simulink model "HMI_2L_StMdXX_Rsp"  (R2018b)
settings: Solver=FixedStepDiscrete  StartTime=0.0  StopTime=10.0  FixedStep=0.01  RelTol=1e-3
undefined symbols (not defined in the file or in its folder): KeSMSuRspStatHldTm_Val, SrcReqTp1
libraries: RspLib x20
(part 1 of 2)
settings Model: Creator=sn2xws  LastModifiedBy=sn2xws
settings DataIOCC: SaveFormat=StructureWithTime
settings OptimizationCC: DefaultParameterBehavior=Inlined  EnhancedBackFolding=on  PassReuseOutputArgsAs=Individual arguments  ZeroExternalMemoryAtStartup=off  ZeroInternalMemoryAtStartup=off  OptimizeBlockOrder=speed  DifferentSizesBufferReuse=on  OptimizationCustomize=off
settings DebuggingCC: ParameterTunabilityLossMsg=error
settings ModelReferenceCC: ModelReferenceNumInstancesAllowed=Single
settings SFSimCC: MATLABDynamicMemAlloc=off
settings RTWCC: SystemTargetFile=autosar.tlc  GenCodeOnly=on  TemplateMakefile=ert_default_tmf  Description=AUTOSAR  GenerateReport=on  IncludeHyperlinkInReport=on  LaunchReport=on  GenerateTraceInfo=on  GenerateTraceReport=on  GenerateTraceReportSl=on  GenerateTraceReportSf=on  GenerateTraceReportEml=on
settings CodeAppCC: ForceParamTrailComments=on  IgnoreCustomStorageClasses=off  OperatorAnnotations=on  SimulinkDataObjDesc=on  SFDataObjDesc=on  InsertBlockDesc=on
settings STFCustomTargetCC: TargetLangStandard=C99 (ISO)  MultiwordLength=256  ParMdlRefBuildCompliant=on  CompOptLevelCompliant=on  IncludeMdlTerminateFcn=off  CombineOutputUpdateFcns=on  SuppressErrorStatus=on  ERTCustomFileBanners=on  SupportNonFinite=off  SupportComplex=off  SupportContinuousTime=off  SupportNonInlinedSFcns=off  RemoveResetFunc=on  MATLABClassNameForMDSCustomization=Simulink.SoftwareTarget.ERTCustomization  AutosarCompliant=on  UseToolchainInfoCompliant=on  LookupTableObjectStructAxisOrder=2,1,3,4,...  LUTObjectStructOrderEvenSpacing=Size,Table,Breakpoints  SystemTargetFile=autosar.tlc
settings ERTTargetCC: TargetLangStandard=C99 (ISO)  ConcurrentExecutionCompliant=off  IncludeMdlTerminateFcn=off  SuppressErrorStatus=on  SupportNonFinite=off  SupportComplex=off  ModelStepFunctionPrototypeControlCompliant=off  CPPClassGenCompliant=off  AutosarCompliant=on  LookupTableObjectStructAxisOrder=2,1,3,4,...  LUTObjectStructOrderEvenSpacing=Size,Table,Breakpoints  InlinedParameterPlacement=NonHierarchical  ERTCustomFileTemplate=example_file_process.tlc

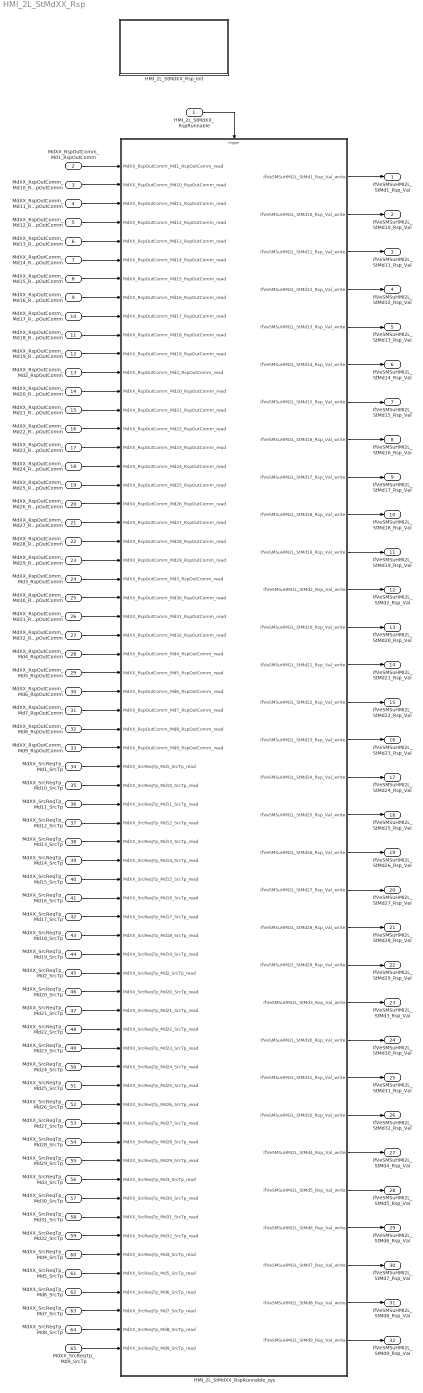
== system HMI_2L_StMdXX_Rsp ==
  HMI_2L_StMdXX_RspRunnable : Inport  SampleTime=0.01  OutputFunctionCall=on
  MdXX_RspOutComm_Md1_RspOutComm : Inport  Port=2  OutDataTypeStr=uint8  PortDimensions=1
  MdXX_RspOutComm_Md10_RspOutComm : Inport  Port=3  OutDataTypeStr=uint8  PortDimensions=1
  MdXX_RspOutComm_Md11_RspOutComm : Inport  Port=4  OutDataTypeStr=uint8  PortDimensions=1
  MdXX_RspOutComm_Md12_RspOutComm : Inport  Port=5  OutDataTypeStr=uint8  PortDimensions=1
  MdXX_RspOutComm_Md13_RspOutComm : Inport  Port=6  OutDataTypeStr=uint8  PortDimensions=1
  MdXX_RspOutComm_Md14_RspOutComm : Inport  Port=7  OutDataTypeStr=uint8  PortDimensions=1
  MdXX_RspOutComm_Md15_RspOutComm : Inport  Port=8  OutDataTypeStr=uint8  PortDimensions=1
  MdXX_RspOutComm_Md16_RspOutComm : Inport  Port=9  OutDataTypeStr=uint8  PortDimensions=1
  MdXX_RspOutComm_Md17_RspOutComm : Inport  Port=10  OutDataTypeStr=uint8  PortDimensions=1
  MdXX_RspOutComm_Md18_RspOutComm : Inport  Port=11  OutDataTypeStr=uint8  PortDimensions=1
  MdXX_RspOutComm_Md19_RspOutComm : Inport  Port=12  OutDataTypeStr=uint8  PortDimensions=1
  MdXX_RspOutComm_Md2_RspOutComm : Inport  Port=13  OutDataTypeStr=uint8  PortDimensions=1
  MdXX_RspOutComm_Md20_RspOutComm : Inport  Port=14  OutDataTypeStr=uint8  PortDimensions=1
  MdXX_RspOutComm_Md21_RspOutComm : Inport  Port=15  OutDataTypeStr=uint8  PortDimensions=1
  MdXX_RspOutComm_Md22_RspOutComm : Inport  Port=16  OutDataTypeStr=uint8  PortDimensions=1
  MdXX_RspOutComm_Md23_RspOutComm : Inport  Port=17  OutDataTypeStr=uint8  PortDimensions=1
  MdXX_RspOutComm_Md24_RspOutComm : Inport  Port=18  OutDataTypeStr=uint8  PortDimensions=1
  MdXX_RspOutComm_Md25_RspOutComm : Inport  Port=19  OutDataTypeStr=uint8  PortDimensions=1
  MdXX_RspOutComm_Md26_RspOutComm : Inport  Port=20  OutDataTypeStr=uint8  PortDimensions=1
  MdXX_RspOutComm_Md27_RspOutComm : Inport  Port=21  OutDataTypeStr=uint8  PortDimensions=1
  MdXX_RspOutComm_Md28_RspOutComm : Inport  Port=22  OutDataTypeStr=uint8  PortDimensions=1
  MdXX_RspOutComm_Md29_RspOutComm : Inport  Port=23  OutDataTypeStr=uint8  PortDimensions=1
  MdXX_RspOutComm_Md3_RspOutComm : Inport  Port=24  OutDataTypeStr=uint8  PortDimensions=1
  MdXX_RspOutComm_Md30_RspOutComm : Inport  Port=25  OutDataTypeStr=uint8  PortDimensions=1
  MdXX_RspOutComm_Md31_RspOutComm : Inport  Port=26  OutDataTypeStr=uint8  PortDimensions=1
  MdXX_RspOutComm_Md32_RspOutComm : Inport  Port=27  OutDataTypeStr=uint8  PortDimensions=1
  MdXX_RspOutComm_Md4_RspOutComm : Inport  Port=28  OutDataTypeStr=uint8  PortDimensions=1
  MdXX_RspOutComm_Md5_RspOutComm : Inport  Port=29  OutDataTypeStr=uint8  PortDimensions=1
  MdXX_RspOutComm_Md6_RspOutComm : Inport  Port=30  OutDataTypeStr=uint8  PortDimensions=1
  MdXX_RspOutComm_Md7_RspOutComm : Inport  Port=31  OutDataTypeStr=uint8  PortDimensions=1
  MdXX_RspOutComm_Md8_RspOutComm : Inport  Port=32  OutDataTypeStr=uint8  PortDimensions=1
  MdXX_RspOutComm_Md9_RspOutComm : Inport  Port=33  OutDataTypeStr=uint8  PortDimensions=1
  MdXX_SrcReqTp_Md1_SrcTp : Inport  Port=34  OutDataTypeStr=Enum: SrcReqTp1  PortDimensions=1
  MdXX_SrcReqTp_Md10_SrcTp : Inport  Port=35  OutDataTypeStr=Enum: SrcReqTp1  PortDimensions=1
  MdXX_SrcReqTp_Md11_SrcTp : Inport  Port=36  OutDataTypeStr=Enum: SrcReqTp1  PortDimensions=1
  MdXX_SrcReqTp_Md12_SrcTp : Inport  Port=37  OutDataTypeStr=Enum: SrcReqTp1  PortDimensions=1
  MdXX_SrcReqTp_Md13_SrcTp : Inport  Port=38  OutDataTypeStr=Enum: SrcReqTp1  PortDimensions=1
  MdXX_SrcReqTp_Md14_SrcTp : Inport  Port=39  OutDataTypeStr=Enum: SrcReqTp1  PortDimensions=1
  MdXX_SrcReqTp_Md15_SrcTp : Inport  Port=40  OutDataTypeStr=Enum: SrcReqTp1  PortDimensions=1
  MdXX_SrcReqTp_Md16_SrcTp : Inport  Port=41  OutDataTypeStr=Enum: SrcReqTp1  PortDimensions=1
  MdXX_SrcReqTp_Md17_SrcTp : Inport  Port=42  OutDataTypeStr=Enum: SrcReqTp1  PortDimensions=1
  MdXX_SrcReqTp_Md18_SrcTp : Inport  Port=43  OutDataTypeStr=Enum: SrcReqTp1  PortDimensions=1
  MdXX_SrcReqTp_Md19_SrcTp : Inport  Port=44  OutDataTypeStr=Enum: SrcReqTp1  PortDimensions=1
  MdXX_SrcReqTp_Md2_SrcTp : Inport  Port=45  OutDataTypeStr=Enum: SrcReqTp1  PortDimensions=1
  MdXX_SrcReqTp_Md20_SrcTp : Inport  Port=46  OutDataTypeStr=Enum: SrcReqTp1  PortDimensions=1
  MdXX_SrcReqTp_Md21_SrcTp : Inport  Port=47  OutDataTypeStr=Enum: SrcReqTp1  PortDimensions=1
  MdXX_SrcReqTp_Md22_SrcTp : Inport  Port=48  OutDataTypeStr=Enum: SrcReqTp1  PortDimensions=1
  MdXX_SrcReqTp_Md23_SrcTp : Inport  Port=49  OutDataTypeStr=Enum: SrcReqTp1  PortDimensions=1
  MdXX_SrcReqTp_Md24_SrcTp : Inport  Port=50  OutDataTypeStr=Enum: SrcReqTp1  PortDimensions=1
  MdXX_SrcReqTp_Md25_SrcTp : Inport  Port=51  OutDataTypeStr=Enum: SrcReqTp1  PortDimensions=1
  MdXX_SrcReqTp_Md26_SrcTp : Inport  Port=52  OutDataTypeStr=Enum: SrcReqTp1  PortDimensions=1
  MdXX_SrcReqTp_Md27_SrcTp : Inport  Port=53  OutDataTypeStr=Enum: SrcReqTp1  PortDimensions=1
  MdXX_SrcReqTp_Md28_SrcTp : Inport  Port=54  OutDataTypeStr=Enum: SrcReqTp1  PortDimensions=1
  MdXX_SrcReqTp_Md29_SrcTp : Inport  Port=55  OutDataTypeStr=Enum: SrcReqTp1  PortDimensions=1
  MdXX_SrcReqTp_Md3_SrcTp : Inport  Port=56  OutDataTypeStr=Enum: SrcReqTp1  PortDimensions=1
  MdXX_SrcReqTp_Md30_SrcTp : Inport  Port=57  OutDataTypeStr=Enum: SrcReqTp1  PortDimensions=1
  MdXX_SrcReqTp_Md31_SrcTp : Inport  Port=58  OutDataTypeStr=Enum: SrcReqTp1  PortDimensions=1
  MdXX_SrcReqTp_Md32_SrcTp : Inport  Port=59  OutDataTypeStr=Enum: SrcReqTp1  PortDimensions=1
  MdXX_SrcReqTp_Md4_SrcTp : Inport  Port=60  OutDataTypeStr=Enum: SrcReqTp1  PortDimensions=1
  MdXX_SrcReqTp_Md5_SrcTp : Inport  Port=61  OutDataTypeStr=Enum: SrcReqTp1  PortDimensions=1
  MdXX_SrcReqTp_Md6_SrcTp : Inport  Port=62  OutDataTypeStr=Enum: SrcReqTp1  PortDimensions=1
  MdXX_SrcReqTp_Md7_SrcTp : Inport  Port=63  OutDataTypeStr=Enum: SrcReqTp1  PortDimensions=1
  MdXX_SrcReqTp_Md8_SrcTp : Inport  Port=64  OutDataTypeStr=Enum: SrcReqTp1  PortDimensions=1
  MdXX_SrcReqTp_Md9_SrcTp : Inport  Port=65  OutDataTypeStr=Enum: SrcReqTp1  PortDimensions=1
  HMI_2L_StMdXX_RspRunnable_sys : Subsystem
  HMI_2L_StMdXX_Rsp_Init : Subsystem
  IfVeSMSuHMI2L_StMd1_Rsp_Val : Outport  OutDataTypeStr=uint8  PortDimensions=1
  IfVeSMSuHMI2L_StMd10_Rsp_Val : Outport  Port=2  OutDataTypeStr=uint8  PortDimensions=1
  IfVeSMSuHMI2L_StMd11_Rsp_Val : Outport  Port=3  OutDataTypeStr=uint8  PortDimensions=1
  IfVeSMSuHMI2L_StMd12_Rsp_Val : Outport  Port=4  OutDataTypeStr=uint8  PortDimensions=1
  IfVeSMSuHMI2L_StMd13_Rsp_Val : Outport  Port=5  OutDataTypeStr=uint8  PortDimensions=1
  IfVeSMSuHMI2L_StMd14_Rsp_Val : Outport  Port=6  OutDataTypeStr=uint8  PortDimensions=1
  IfVeSMSuHMI2L_StMd15_Rsp_Val : Outport  Port=7  OutDataTypeStr=uint8  PortDimensions=1
  IfVeSMSuHMI2L_StMd16_Rsp_Val : Outport  Port=8  OutDataTypeStr=uint8  PortDimensions=1
  IfVeSMSuHMI2L_StMd17_Rsp_Val : Outport  Port=9  OutDataTypeStr=uint8  PortDimensions=1
  IfVeSMSuHMI2L_StMd18_Rsp_Val : Outport  Port=10  OutDataTypeStr=uint8  PortDimensions=1
  IfVeSMSuHMI2L_StMd19_Rsp_Val : Outport  Port=11  OutDataTypeStr=uint8  PortDimensions=1
  IfVeSMSuHMI2L_StMd2_Rsp_Val : Outport  Port=12  OutDataTypeStr=uint8  PortDimensions=1
  IfVeSMSuHMI2L_StMd20_Rsp_Val : Outport  Port=13  OutDataTypeStr=uint8  PortDimensions=1
  IfVeSMSuHMI2L_StMd21_Rsp_Val : Outport  Port=14  OutDataTypeStr=uint8  PortDimensions=1
  IfVeSMSuHMI2L_StMd22_Rsp_Val : Outport  Port=15  OutDataTypeStr=uint8  PortDimensions=1
  IfVeSMSuHMI2L_StMd23_Rsp_Val : Outport  Port=16  OutDataTypeStr=uint8  PortDimensions=1
  IfVeSMSuHMI2L_StMd24_Rsp_Val : Outport  Port=17  OutDataTypeStr=uint8  PortDimensions=1
  IfVeSMSuHMI2L_StMd25_Rsp_Val : Outport  Port=18  OutDataTypeStr=uint8  PortDimensions=1
  IfVeSMSuHMI2L_StMd26_Rsp_Val : Outport  Port=19  OutDataTypeStr=uint8  PortDimensions=1
  IfVeSMSuHMI2L_StMd27_Rsp_Val : Outport  Port=20  OutDataTypeStr=uint8  PortDimensions=1
  IfVeSMSuHMI2L_StMd28_Rsp_Val : Outport  Port=21  OutDataTypeStr=uint8  PortDimensions=1
  IfVeSMSuHMI2L_StMd29_Rsp_Val : Outport  Port=22  OutDataTypeStr=uint8  PortDimensions=1
  IfVeSMSuHMI2L_StMd3_Rsp_Val : Outport  Port=23  OutDataTypeStr=uint8  PortDimensions=1
  IfVeSMSuHMI2L_StMd30_Rsp_Val : Outport  Port=24  OutDataTypeStr=uint8  PortDimensions=1
  IfVeSMSuHMI2L_StMd31_Rsp_Val : Outport  Port=25  OutDataTypeStr=uint8  PortDimensions=1
  IfVeSMSuHMI2L_StMd32_Rsp_Val : Outport  Port=26  OutDataTypeStr=uint8  PortDimensions=1
  IfVeSMSuHMI2L_StMd4_Rsp_Val : Outport  Port=27  OutDataTypeStr=uint8  PortDimensions=1
  IfVeSMSuHMI2L_StMd5_Rsp_Val : Outport  Port=28  OutDataTypeStr=uint8  PortDimensions=1
  IfVeSMSuHMI2L_StMd6_Rsp_Val : Outport  Port=29  OutDataTypeStr=uint8  PortDimensions=1
  IfVeSMSuHMI2L_StMd7_Rsp_Val : Outport  Port=30  OutDataTypeStr=uint8  PortDimensions=1
  IfVeSMSuHMI2L_StMd8_Rsp_Val : Outport  Port=31  OutDataTypeStr=uint8  PortDimensions=1
  IfVeSMSuHMI2L_StMd9_Rsp_Val : Outport  Port=32  OutDataTypeStr=uint8  PortDimensions=1
  wires:
  MdXX_RspOutComm_Md1_RspOutComm/1 -> HMI_2L_StMdXX_RspRunnable_sys/1(MdXX_RspOutComm_Md1_RspOutComm_read)
  MdXX_RspOutComm_Md10_RspOutComm/1 -> HMI_2L_StMdXX_RspRunnable_sys/2(MdXX_RspOutComm_Md10_RspOutComm_read)
  MdXX_RspOutComm_Md11_RspOutComm/1 -> HMI_2L_StMdXX_RspRunnable_sys/3(MdXX_RspOutComm_Md11_RspOutComm_read)
  MdXX_RspOutComm_Md12_RspOutComm/1 -> HMI_2L_StMdXX_RspRunnable_sys/4(MdXX_RspOutComm_Md12_RspOutComm_read)
  MdXX_RspOutComm_Md13_RspOutComm/1 -> HMI_2L_StMdXX_RspRunnable_sys/5(MdXX_RspOutComm_Md13_RspOutComm_read)
  MdXX_RspOutComm_Md14_RspOutComm/1 -> HMI_2L_StMdXX_RspRunnable_sys/6(MdXX_RspOutComm_Md14_RspOutComm_read)
  MdXX_RspOutComm_Md15_RspOutComm/1 -> HMI_2L_StMdXX_RspRunnable_sys/7(MdXX_RspOutComm_Md15_RspOutComm_read)
  MdXX_RspOutComm_Md16_RspOutComm/1 -> HMI_2L_StMdXX_RspRunnable_sys/8(MdXX_RspOutComm_Md16_RspOutComm_read)
  MdXX_RspOutComm_Md17_RspOutComm/1 -> HMI_2L_StMdXX_RspRunnable_sys/9(MdXX_RspOutComm_Md17_RspOutComm_read)
  MdXX_RspOutComm_Md18_RspOutComm/1 -> HMI_2L_StMdXX_RspRunnable_sys/10(MdXX_RspOutComm_Md18_RspOutComm_read)
  MdXX_RspOutComm_Md19_RspOutComm/1 -> HMI_2L_StMdXX_RspRunnable_sys/11(MdXX_RspOutComm_Md19_RspOutComm_read)
  MdXX_RspOutComm_Md2_RspOutComm/1 -> HMI_2L_StMdXX_RspRunnable_sys/12(MdXX_RspOutComm_Md2_RspOutComm_read)
  MdXX_RspOutComm_Md20_RspOutComm/1 -> HMI_2L_StMdXX_RspRunnable_sys/13(MdXX_RspOutComm_Md20_RspOutComm_read)
  MdXX_RspOutComm_Md21_RspOutComm/1 -> HMI_2L_StMdXX_RspRunnable_sys/14(MdXX_RspOutComm_Md21_RspOutComm_read)
  MdXX_RspOutComm_Md22_RspOutComm/1 -> HMI_2L_StMdXX_RspRunnable_sys/15(MdXX_RspOutComm_Md22_RspOutComm_read)
  MdXX_RspOutComm_Md23_RspOutComm/1 -> HMI_2L_StMdXX_RspRunnable_sys/16(MdXX_RspOutComm_Md23_RspOutComm_read)
  MdXX_RspOutComm_Md24_RspOutComm/1 -> HMI_2L_StMdXX_RspRunnable_sys/17(MdXX_RspOutComm_Md24_RspOutComm_read)
  MdXX_RspOutComm_Md25_RspOutComm/1 -> HMI_2L_StMdXX_RspRunnable_sys/18(MdXX_RspOutComm_Md25_RspOutComm_read)
  MdXX_RspOutComm_Md26_RspOutComm/1 -> HMI_2L_StMdXX_RspRunnable_sys/19(MdXX_RspOutComm_Md26_RspOutComm_read)
  MdXX_RspOutComm_Md27_RspOutComm/1 -> HMI_2L_StMdXX_RspRunnable_sys/20(MdXX_RspOutComm_Md27_RspOutComm_read)
  MdXX_RspOutComm_Md28_RspOutComm/1 -> HMI_2L_StMdXX_RspRunnable_sys/21(MdXX_RspOutComm_Md28_RspOutComm_read)
  MdXX_RspOutComm_Md29_RspOutComm/1 -> HMI_2L_StMdXX_RspRunnable_sys/22(MdXX_RspOutComm_Md29_RspOutComm_read)
  MdXX_RspOutComm_Md3_RspOutComm/1 -> HMI_2L_StMdXX_RspRunnable_sys/23(MdXX_RspOutComm_Md3_RspOutComm_read)
  MdXX_RspOutComm_Md30_RspOutComm/1 -> HMI_2L_StMdXX_RspRunnable_sys/24(MdXX_RspOutComm_Md30_RspOutComm_read)
  MdXX_RspOutComm_Md31_RspOutComm/1 -> HMI_2L_StMdXX_RspRunnable_sys/25(MdXX_RspOutComm_Md31_RspOutComm_read)
  MdXX_RspOutComm_Md32_RspOutComm/1 -> HMI_2L_StMdXX_RspRunnable_sys/26(MdXX_RspOutComm_Md32_RspOutComm_read)
  MdXX_RspOutComm_Md4_RspOutComm/1 -> HMI_2L_StMdXX_RspRunnable_sys/27(MdXX_RspOutComm_Md4_RspOutComm_read)
  MdXX_RspOutComm_Md5_RspOutComm/1 -> HMI_2L_StMdXX_RspRunnable_sys/28(MdXX_RspOutComm_Md5_RspOutComm_read)
  MdXX_RspOutComm_Md6_RspOutComm/1 -> HMI_2L_StMdXX_RspRunnable_sys/29(MdXX_RspOutComm_Md6_RspOutComm_read)
  MdXX_RspOutComm_Md7_RspOutComm/1 -> HMI_2L_StMdXX_RspRunnable_sys/30(MdXX_RspOutComm_Md7_RspOutComm_read)
  MdXX_RspOutComm_Md8_RspOutComm/1 -> HMI_2L_StMdXX_RspRunnable_sys/31(MdXX_RspOutComm_Md8_RspOutComm_read)
  MdXX_RspOutComm_Md9_RspOutComm/1 -> HMI_2L_StMdXX_RspRunnable_sys/32(MdXX_RspOutComm_Md9_RspOutComm_read)
  MdXX_SrcReqTp_Md1_SrcTp/1 -> HMI_2L_StMdXX_RspRunnable_sys/33(MdXX_SrcReqTp_Md1_SrcTp_read)
  MdXX_SrcReqTp_Md10_SrcTp/1 -> HMI_2L_StMdXX_RspRunnable_sys/34(MdXX_SrcReqTp_Md10_SrcTp_read)
  MdXX_SrcReqTp_Md11_SrcTp/1 -> HMI_2L_StMdXX_RspRunnable_sys/35(MdXX_SrcReqTp_Md11_SrcTp_read)
  MdXX_SrcReqTp_Md12_SrcTp/1 -> HMI_2L_StMdXX_RspRunnable_sys/36(MdXX_SrcReqTp_Md12_SrcTp_read)
  MdXX_SrcReqTp_Md13_SrcTp/1 -> HMI_2L_StMdXX_RspRunnable_sys/37(MdXX_SrcReqTp_Md13_SrcTp_read)
  MdXX_SrcReqTp_Md14_SrcTp/1 -> HMI_2L_StMdXX_RspRunnable_sys/38(MdXX_SrcReqTp_Md14_SrcTp_read)
  MdXX_SrcReqTp_Md15_SrcTp/1 -> HMI_2L_StMdXX_RspRunnable_sys/39(MdXX_SrcReqTp_Md15_SrcTp_read)
  MdXX_SrcReqTp_Md16_SrcTp/1 -> HMI_2L_StMdXX_RspRunnable_sys/40(MdXX_SrcReqTp_Md16_SrcTp_read)
  MdXX_SrcReqTp_Md17_SrcTp/1 -> HMI_2L_StMdXX_RspRunnable_sys/41(MdXX_SrcReqTp_Md17_SrcTp_read)
  MdXX_SrcReqTp_Md18_SrcTp/1 -> HMI_2L_StMdXX_RspRunnable_sys/42(MdXX_SrcReqTp_Md18_SrcTp_read)
  MdXX_SrcReqTp_Md19_SrcTp/1 -> HMI_2L_StMdXX_RspRunnable_sys/43(MdXX_SrcReqTp_Md19_SrcTp_read)
  MdXX_SrcReqTp_Md2_SrcTp/1 -> HMI_2L_StMdXX_RspRunnable_sys/44(MdXX_SrcReqTp_Md2_SrcTp_read)
  MdXX_SrcReqTp_Md20_SrcTp/1 -> HMI_2L_StMdXX_RspRunnable_sys/45(MdXX_SrcReqTp_Md20_SrcTp_read)
  MdXX_SrcReqTp_Md21_SrcTp/1 -> HMI_2L_StMdXX_RspRunnable_sys/46(MdXX_SrcReqTp_Md21_SrcTp_read)
  MdXX_SrcReqTp_Md22_SrcTp/1 -> HMI_2L_StMdXX_RspRunnable_sys/47(MdXX_SrcReqTp_Md22_SrcTp_read)
  MdXX_SrcReqTp_Md23_SrcTp/1 -> HMI_2L_StMdXX_RspRunnable_sys/48(MdXX_SrcReqTp_Md23_SrcTp_read)
  MdXX_SrcReqTp_Md24_SrcTp/1 -> HMI_2L_StMdXX_RspRunnable_sys/49(MdXX_SrcReqTp_Md24_SrcTp_read)
  MdXX_SrcReqTp_Md25_SrcTp/1 -> HMI_2L_StMdXX_RspRunnable_sys/50(MdXX_SrcReqTp_Md25_SrcTp_read)
  MdXX_SrcReqTp_Md26_SrcTp/1 -> HMI_2L_StMdXX_RspRunnable_sys/51(MdXX_SrcReqTp_Md26_SrcTp_read)
  MdXX_SrcReqTp_Md27_SrcTp/1 -> HMI_2L_StMdXX_RspRunnable_sys/52(MdXX_SrcReqTp_Md27_SrcTp_read)
  MdXX_SrcReqTp_Md28_SrcTp/1 -> HMI_2L_StMdXX_RspRunnable_sys/53(MdXX_SrcReqTp_Md28_SrcTp_read)
  MdXX_SrcReqTp_Md29_SrcTp/1 -> HMI_2L_StMdXX_RspRunnable_sys/54(MdXX_SrcReqTp_Md29_SrcTp_read)
  MdXX_SrcReqTp_Md3_SrcTp/1 -> HMI_2L_StMdXX_RspRunnable_sys/55(MdXX_SrcReqTp_Md3_SrcTp_read)
  MdXX_SrcReqTp_Md30_SrcTp/1 -> HMI_2L_StMdXX_RspRunnable_sys/56(MdXX_SrcReqTp_Md30_SrcTp_read)
  MdXX_SrcReqTp_Md31_SrcTp/1 -> HMI_2L_StMdXX_RspRunnable_sys/57(MdXX_SrcReqTp_Md31_SrcTp_read)
  MdXX_SrcReqTp_Md32_SrcTp/1 -> HMI_2L_StMdXX_RspRunnable_sys/58(MdXX_SrcReqTp_Md32_SrcTp_read)
  MdXX_SrcReqTp_Md4_SrcTp/1 -> HMI_2L_StMdXX_RspRunnable_sys/59(MdXX_SrcReqTp_Md4_SrcTp_read)
  MdXX_SrcReqTp_Md5_SrcTp/1 -> HMI_2L_StMdXX_RspRunnable_sys/60(MdXX_SrcReqTp_Md5_SrcTp_read)
  MdXX_SrcReqTp_Md6_SrcTp/1 -> HMI_2L_StMdXX_RspRunnable_sys/61(MdXX_SrcReqTp_Md6_SrcTp_read)
  MdXX_SrcReqTp_Md7_SrcTp/1 -> HMI_2L_StMdXX_RspRunnable_sys/62(MdXX_SrcReqTp_Md7_SrcTp_read)
  MdXX_SrcReqTp_Md8_SrcTp/1 -> HMI_2L_StMdXX_RspRunnable_sys/63(MdXX_SrcReqTp_Md8_SrcTp_read)
  MdXX_SrcReqTp_Md9_SrcTp/1 -> HMI_2L_StMdXX_RspRunnable_sys/64(MdXX_SrcReqTp_Md9_SrcTp_read)
  HMI_2L_StMdXX_RspRunnable_sys/1(IfVeSMSuHMI2L_StMd1_Rsp_Val_write) -> IfVeSMSuHMI2L_StMd1_Rsp_Val/1
  HMI_2L_StMdXX_RspRunnable_sys/2(IfVeSMSuHMI2L_StMd10_Rsp_Val_write) -> IfVeSMSuHMI2L_StMd10_Rsp_Val/1
  HMI_2L_StMdXX_RspRunnable_sys/3(IfVeSMSuHMI2L_StMd11_Rsp_Val_write) -> IfVeSMSuHMI2L_StMd11_Rsp_Val/1
  HMI_2L_StMdXX_RspRunnable_sys/4(IfVeSMSuHMI2L_StMd12_Rsp_Val_write) -> IfVeSMSuHMI2L_StMd12_Rsp_Val/1
  HMI_2L_StMdXX_RspRunnable_sys/5(IfVeSMSuHMI2L_StMd13_Rsp_Val_write) -> IfVeSMSuHMI2L_StMd13_Rsp_Val/1
  HMI_2L_StMdXX_RspRunnable_sys/6(IfVeSMSuHMI2L_StMd14_Rsp_Val_write) -> IfVeSMSuHMI2L_StMd14_Rsp_Val/1
  HMI_2L_StMdXX_RspRunnable_sys/7(IfVeSMSuHMI2L_StMd15_Rsp_Val_write) -> IfVeSMSuHMI2L_StMd15_Rsp_Val/1
  HMI_2L_StMdXX_RspRunnable_sys/8(IfVeSMSuHMI2L_StMd16_Rsp_Val_write) -> IfVeSMSuHMI2L_StMd16_Rsp_Val/1
  HMI_2L_StMdXX_RspRunnable_sys/9(IfVeSMSuHMI2L_StMd17_Rsp_Val_write) -> IfVeSMSuHMI2L_StMd17_Rsp_Val/1
  HMI_2L_StMdXX_RspRunnable_sys/10(IfVeSMSuHMI2L_StMd18_Rsp_Val_write) -> IfVeSMSuHMI2L_StMd18_Rsp_Val/1
  HMI_2L_StMdXX_RspRunnable_sys/11(IfVeSMSuHMI2L_StMd19_Rsp_Val_write) -> IfVeSMSuHMI2L_StMd19_Rsp_Val/1
  HMI_2L_StMdXX_RspRunnable_sys/12(IfVeSMSuHMI2L_StMd2_Rsp_Val_write) -> IfVeSMSuHMI2L_StMd2_Rsp_Val/1
  HMI_2L_StMdXX_RspRunnable_sys/13(IfVeSMSuHMI2L_StMd20_Rsp_Val_write) -> IfVeSMSuHMI2L_StMd20_Rsp_Val/1
  HMI_2L_StMdXX_RspRunnable_sys/14(IfVeSMSuHMI2L_StMd21_Rsp_Val_write) -> IfVeSMSuHMI2L_StMd21_Rsp_Val/1
  HMI_2L_StMdXX_RspRunnable_sys/15(IfVeSMSuHMI2L_StMd22_Rsp_Val_write) -> IfVeSMSuHMI2L_StMd22_Rsp_Val/1
  HMI_2L_StMdXX_RspRunnable_sys/16(IfVeSMSuHMI2L_StMd23_Rsp_Val_write) -> IfVeSMSuHMI2L_StMd23_Rsp_Val/1
  HMI_2L_StMdXX_RspRunnable_sys/17(IfVeSMSuHMI2L_StMd24_Rsp_Val_write) -> IfVeSMSuHMI2L_StMd24_Rsp_Val/1
  HMI_2L_StMdXX_RspRunnable_sys/18(IfVeSMSuHMI2L_StMd25_Rsp_Val_write) -> IfVeSMSuHMI2L_StMd25_Rsp_Val/1
  HMI_2L_StMdXX_RspRunnable_sys/19(IfVeSMSuHMI2L_StMd26_Rsp_Val_write) -> IfVeSMSuHMI2L_StMd26_Rsp_Val/1
  HMI_2L_StMdXX_RspRunnable_sys/20(IfVeSMSuHMI2L_StMd27_Rsp_Val_write) -> IfVeSMSuHMI2L_StMd27_Rsp_Val/1
  HMI_2L_StMdXX_RspRunnable_sys/21(IfVeSMSuHMI2L_StMd28_Rsp_Val_write) -> IfVeSMSuHMI2L_StMd28_Rsp_Val/1
  HMI_2L_StMdXX_RspRunnable_sys/22(IfVeSMSuHMI2L_StMd29_Rsp_Val_write) -> IfVeSMSuHMI2L_StMd29_Rsp_Val/1
  HMI_2L_StMdXX_RspRunnable_sys/23(IfVeSMSuHMI2L_StMd3_Rsp_Val_write) -> IfVeSMSuHMI2L_StMd3_Rsp_Val/1
  HMI_2L_StMdXX_RspRunnable_sys/24(IfVeSMSuHMI2L_StMd30_Rsp_Val_write) -> IfVeSMSuHMI2L_StMd30_Rsp_Val/1
  HMI_2L_StMdXX_RspRunnable_sys/25(IfVeSMSuHMI2L_StMd31_Rsp_Val_write) -> IfVeSMSuHMI2L_StMd31_Rsp_Val/1
  HMI_2L_StMdXX_RspRunnable_sys/26(IfVeSMSuHMI2L_StMd32_Rsp_Val_write) -> IfVeSMSuHMI2L_StMd32_Rsp_Val/1
  HMI_2L_StMdXX_RspRunnable_sys/27(IfVeSMSuHMI2L_StMd4_Rsp_Val_write) -> IfVeSMSuHMI2L_StMd4_Rsp_Val/1
  HMI_2L_StMdXX_RspRunnable_sys/28(IfVeSMSuHMI2L_StMd5_Rsp_Val_write) -> IfVeSMSuHMI2L_StMd5_Rsp_Val/1
  HMI_2L_StMdXX_RspRunnable_sys/29(IfVeSMSuHMI2L_StMd6_Rsp_Val_write) -> IfVeSMSuHMI2L_StMd6_Rsp_Val/1
  HMI_2L_StMdXX_RspRunnable_sys/30(IfVeSMSuHMI2L_StMd7_Rsp_Val_write) -> IfVeSMSuHMI2L_StMd7_Rsp_Val/1
  HMI_2L_StMdXX_RspRunnable_sys/31(IfVeSMSuHMI2L_StMd8_Rsp_Val_write) -> IfVeSMSuHMI2L_StMd8_Rsp_Val/1
  HMI_2L_StMdXX_RspRunnable_sys/32(IfVeSMSuHMI2L_StMd9_Rsp_Val_write) -> IfVeSMSuHMI2L_StMd9_Rsp_Val/1
  HMI_2L_StMdXX_RspRunnable/1 -> HMI_2L_StMdXX_RspRunnable_sys/Trigger

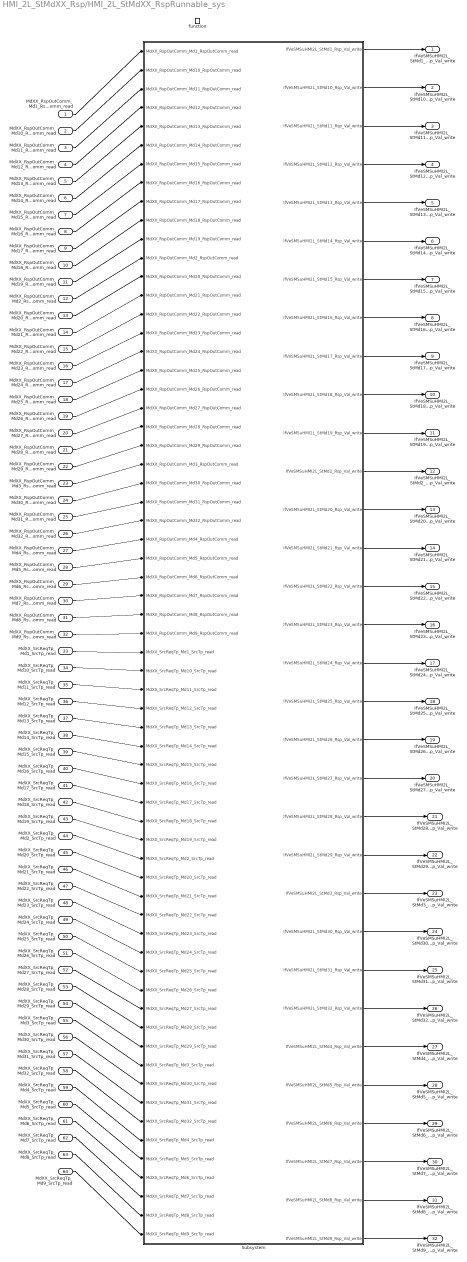
== system HMI_2L_StMdXX_Rsp/HMI_2L_StMdXX_RspRunnable_sys ==
  MdXX_RspOutComm_Md1_RspOutComm_read : Inport
  MdXX_RspOutComm_Md10_RspOutComm_read : Inport  Port=2
  MdXX_RspOutComm_Md11_RspOutComm_read : Inport  Port=3
  MdXX_RspOutComm_Md12_RspOutComm_read : Inport  Port=4
  MdXX_RspOutComm_Md13_RspOutComm_read : Inport  Port=5
  MdXX_RspOutComm_Md14_RspOutComm_read : Inport  Port=6
  MdXX_RspOutComm_Md15_RspOutComm_read : Inport  Port=7
  MdXX_RspOutComm_Md16_RspOutComm_read : Inport  Port=8
  MdXX_RspOutComm_Md17_RspOutComm_read : Inport  Port=9
  MdXX_RspOutComm_Md18_RspOutComm_read : Inport  Port=10
  MdXX_RspOutComm_Md19_RspOutComm_read : Inport  Port=11
  MdXX_RspOutComm_Md2_RspOutComm_read : Inport  Port=12
  MdXX_RspOutComm_Md20_RspOutComm_read : Inport  Port=13
  MdXX_RspOutComm_Md21_RspOutComm_read : Inport  Port=14
  MdXX_RspOutComm_Md22_RspOutComm_read : Inport  Port=15
  MdXX_RspOutComm_Md23_RspOutComm_read : Inport  Port=16
  MdXX_RspOutComm_Md24_RspOutComm_read : Inport  Port=17
  MdXX_RspOutComm_Md25_RspOutComm_read : Inport  Port=18
  MdXX_RspOutComm_Md26_RspOutComm_read : Inport  Port=19
  MdXX_RspOutComm_Md27_RspOutComm_read : Inport  Port=20
  MdXX_RspOutComm_Md28_RspOutComm_read : Inport  Port=21
  MdXX_RspOutComm_Md29_RspOutComm_read : Inport  Port=22
  MdXX_RspOutComm_Md3_RspOutComm_read : Inport  Port=23
  MdXX_RspOutComm_Md30_RspOutComm_read : Inport  Port=24
  MdXX_RspOutComm_Md31_RspOutComm_read : Inport  Port=25
  MdXX_RspOutComm_Md32_RspOutComm_read : Inport  Port=26
  MdXX_RspOutComm_Md4_RspOutComm_read : Inport  Port=27
  MdXX_RspOutComm_Md5_RspOutComm_read : Inport  Port=28
  MdXX_RspOutComm_Md6_RspOutComm_read : Inport  Port=29
  MdXX_RspOutComm_Md7_RspOutComm_read : Inport  Port=30
  MdXX_RspOutComm_Md8_RspOutComm_read : Inport  Port=31
  MdXX_RspOutComm_Md9_RspOutComm_read : Inport  Port=32
  MdXX_SrcReqTp_Md1_SrcTp_read : Inport  Port=33
  MdXX_SrcReqTp_Md10_SrcTp_read : Inport  Port=34
  MdXX_SrcReqTp_Md11_SrcTp_read : Inport  Port=35
  MdXX_SrcReqTp_Md12_SrcTp_read : Inport  Port=36
  MdXX_SrcReqTp_Md13_SrcTp_read : Inport  Port=37
  MdXX_SrcReqTp_Md14_SrcTp_read : Inport  Port=38
  MdXX_SrcReqTp_Md15_SrcTp_read : Inport  Port=39
  MdXX_SrcReqTp_Md16_SrcTp_read : Inport  Port=40
  MdXX_SrcReqTp_Md17_SrcTp_read : Inport  Port=41
  MdXX_SrcReqTp_Md18_SrcTp_read : Inport  Port=42
  MdXX_SrcReqTp_Md19_SrcTp_read : Inport  Port=43
  MdXX_SrcReqTp_Md2_SrcTp_read : Inport  Port=44
  MdXX_SrcReqTp_Md20_SrcTp_read : Inport  Port=45
  MdXX_SrcReqTp_Md21_SrcTp_read : Inport  Port=46
  MdXX_SrcReqTp_Md22_SrcTp_read : Inport  Port=47
  MdXX_SrcReqTp_Md23_SrcTp_read : Inport  Port=48
  MdXX_SrcReqTp_Md24_SrcTp_read : Inport  Port=49
  MdXX_SrcReqTp_Md25_SrcTp_read : Inport  Port=50
  MdXX_SrcReqTp_Md26_SrcTp_read : Inport  Port=51
  MdXX_SrcReqTp_Md27_SrcTp_read : Inport  Port=52
  MdXX_SrcReqTp_Md28_SrcTp_read : Inport  Port=53
  MdXX_SrcReqTp_Md29_SrcTp_read : Inport  Port=54
  MdXX_SrcReqTp_Md3_SrcTp_read : Inport  Port=55
  MdXX_SrcReqTp_Md30_SrcTp_read : Inport  Port=56
  MdXX_SrcReqTp_Md31_SrcTp_read : Inport  Port=57
  MdXX_SrcReqTp_Md32_SrcTp_read : Inport  Port=58
  MdXX_SrcReqTp_Md4_SrcTp_read : Inport  Port=59
  MdXX_SrcReqTp_Md5_SrcTp_read : Inport  Port=60
  MdXX_SrcReqTp_Md6_SrcTp_read : Inport  Port=61
  MdXX_SrcReqTp_Md7_SrcTp_read : Inport  Port=62
  MdXX_SrcReqTp_Md8_SrcTp_read : Inport  Port=63
  MdXX_SrcReqTp_Md9_SrcTp_read : Inport  Port=64
  function : TriggerPort  TriggerType=function-call  VariantControl=(inherit)  SampleTimeType=periodic  SampleTime=-1
  Subsystem : Subsystem
  IfVeSMSuHMI2L_StMd1_Rsp_Val_write : Outport
      settings: EnsureOutportIsVirtual=on
  IfVeSMSuHMI2L_StMd10_Rsp_Val_write : Outport  Port=2
      settings: EnsureOutportIsVirtual=on
  IfVeSMSuHMI2L_StMd11_Rsp_Val_write : Outport  Port=3
      settings: EnsureOutportIsVirtual=on
  IfVeSMSuHMI2L_StMd12_Rsp_Val_write : Outport  Port=4
      settings: EnsureOutportIsVirtual=on
  IfVeSMSuHMI2L_StMd13_Rsp_Val_write : Outport  Port=5
      settings: EnsureOutportIsVirtual=on
  IfVeSMSuHMI2L_StMd14_Rsp_Val_write : Outport  Port=6
      settings: EnsureOutportIsVirtual=on
  IfVeSMSuHMI2L_StMd15_Rsp_Val_write : Outport  Port=7
      settings: EnsureOutportIsVirtual=on
  IfVeSMSuHMI2L_StMd16_Rsp_Val_write : Outport  Port=8
      settings: EnsureOutportIsVirtual=on
  IfVeSMSuHMI2L_StMd17_Rsp_Val_write : Outport  Port=9
      settings: EnsureOutportIsVirtual=on
  IfVeSMSuHMI2L_StMd18_Rsp_Val_write : Outport  Port=10
      settings: EnsureOutportIsVirtual=on
  IfVeSMSuHMI2L_StMd19_Rsp_Val_write : Outport  Port=11
      settings: EnsureOutportIsVirtual=on
  IfVeSMSuHMI2L_StMd2_Rsp_Val_write : Outport  Port=12
      settings: EnsureOutportIsVirtual=on
  IfVeSMSuHMI2L_StMd20_Rsp_Val_write : Outport  Port=13
      settings: EnsureOutportIsVirtual=on
  IfVeSMSuHMI2L_StMd21_Rsp_Val_write : Outport  Port=14
      settings: EnsureOutportIsVirtual=on
  IfVeSMSuHMI2L_StMd22_Rsp_Val_write : Outport  Port=15
      settings: EnsureOutportIsVirtual=on
  IfVeSMSuHMI2L_StMd23_Rsp_Val_write : Outport  Port=16
      settings: EnsureOutportIsVirtual=on
  IfVeSMSuHMI2L_StMd24_Rsp_Val_write : Outport  Port=17
      settings: EnsureOutportIsVirtual=on
  IfVeSMSuHMI2L_StMd25_Rsp_Val_write : Outport  Port=18
      settings: EnsureOutportIsVirtual=on
  IfVeSMSuHMI2L_StMd26_Rsp_Val_write : Outport  Port=19
      settings: EnsureOutportIsVirtual=on
  IfVeSMSuHMI2L_StMd27_Rsp_Val_write : Outport  Port=20
      settings: EnsureOutportIsVirtual=on
  IfVeSMSuHMI2L_StMd28_Rsp_Val_write : Outport  Port=21
      settings: EnsureOutportIsVirtual=on
  IfVeSMSuHMI2L_StMd29_Rsp_Val_write : Outport  Port=22
      settings: EnsureOutportIsVirtual=on
  IfVeSMSuHMI2L_StMd3_Rsp_Val_write : Outport  Port=23
      settings: EnsureOutportIsVirtual=on
  IfVeSMSuHMI2L_StMd30_Rsp_Val_write : Outport  Port=24
      settings: EnsureOutportIsVirtual=on
  IfVeSMSuHMI2L_StMd31_Rsp_Val_write : Outport  Port=25
      settings: EnsureOutportIsVirtual=on
  IfVeSMSuHMI2L_StMd32_Rsp_Val_write : Outport  Port=26
      settings: EnsureOutportIsVirtual=on
  IfVeSMSuHMI2L_StMd4_Rsp_Val_write : Outport  Port=27
      settings: EnsureOutportIsVirtual=on
  IfVeSMSuHMI2L_StMd5_Rsp_Val_write : Outport  Port=28
      settings: EnsureOutportIsVirtual=on
  IfVeSMSuHMI2L_StMd6_Rsp_Val_write : Outport  Port=29
      settings: EnsureOutportIsVirtual=on
  IfVeSMSuHMI2L_StMd7_Rsp_Val_write : Outport  Port=30
      settings: EnsureOutportIsVirtual=on
  IfVeSMSuHMI2L_StMd8_Rsp_Val_write : Outport  Port=31
      settings: EnsureOutportIsVirtual=on
  IfVeSMSuHMI2L_StMd9_Rsp_Val_write : Outport  Port=32
      settings: EnsureOutportIsVirtual=on
  wires:
  MdXX_RspOutComm_Md1_RspOutComm_read/1 -> Subsystem/1(MdXX_RspOutComm_Md1_RspOutComm_read)
  MdXX_RspOutComm_Md10_RspOutComm_read/1 -> Subsystem/2(MdXX_RspOutComm_Md10_RspOutComm_read)
  MdXX_RspOutComm_Md11_RspOutComm_read/1 -> Subsystem/3(MdXX_RspOutComm_Md11_RspOutComm_read)
  MdXX_RspOutComm_Md12_RspOutComm_read/1 -> Subsystem/4(MdXX_RspOutComm_Md12_RspOutComm_read)
  MdXX_RspOutComm_Md13_RspOutComm_read/1 -> Subsystem/5(MdXX_RspOutComm_Md13_RspOutComm_read)
  MdXX_RspOutComm_Md14_RspOutComm_read/1 -> Subsystem/6(MdXX_RspOutComm_Md14_RspOutComm_read)
  MdXX_RspOutComm_Md15_RspOutComm_read/1 -> Subsystem/7(MdXX_RspOutComm_Md15_RspOutComm_read)
  MdXX_RspOutComm_Md16_RspOutComm_read/1 -> Subsystem/8(MdXX_RspOutComm_Md16_RspOutComm_read)
  MdXX_RspOutComm_Md17_RspOutComm_read/1 -> Subsystem/9(MdXX_RspOutComm_Md17_RspOutComm_read)
  MdXX_RspOutComm_Md18_RspOutComm_read/1 -> Subsystem/10(MdXX_RspOutComm_Md18_RspOutComm_read)
  MdXX_RspOutComm_Md19_RspOutComm_read/1 -> Subsystem/11(MdXX_RspOutComm_Md19_RspOutComm_read)
  MdXX_RspOutComm_Md2_RspOutComm_read/1 -> Subsystem/12(MdXX_RspOutComm_Md2_RspOutComm_read)
  MdXX_RspOutComm_Md20_RspOutComm_read/1 -> Subsystem/13(MdXX_RspOutComm_Md20_RspOutComm_read)
  MdXX_RspOutComm_Md21_RspOutComm_read/1 -> Subsystem/14(MdXX_RspOutComm_Md21_RspOutComm_read)
  MdXX_RspOutComm_Md22_RspOutComm_read/1 -> Subsystem/15(MdXX_RspOutComm_Md22_RspOutComm_read)
  MdXX_RspOutComm_Md23_RspOutComm_read/1 -> Subsystem/16(MdXX_RspOutComm_Md23_RspOutComm_read)
  MdXX_RspOutComm_Md24_RspOutComm_read/1 -> Subsystem/17(MdXX_RspOutComm_Md24_RspOutComm_read)
  MdXX_RspOutComm_Md25_RspOutComm_read/1 -> Subsystem/18(MdXX_RspOutComm_Md25_RspOutComm_read)
  MdXX_RspOutComm_Md26_RspOutComm_read/1 -> Subsystem/19(MdXX_RspOutComm_Md26_RspOutComm_read)
  MdXX_RspOutComm_Md27_RspOutComm_read/1 -> Subsystem/20(MdXX_RspOutComm_Md27_RspOutComm_read)
  MdXX_RspOutComm_Md28_RspOutComm_read/1 -> Subsystem/21(MdXX_RspOutComm_Md28_RspOutComm_read)
  MdXX_RspOutComm_Md29_RspOutComm_read/1 -> Subsystem/22(MdXX_RspOutComm_Md29_RspOutComm_read)
  MdXX_RspOutComm_Md3_RspOutComm_read/1 -> Subsystem/23(MdXX_RspOutComm_Md3_RspOutComm_read)
  MdXX_RspOutComm_Md30_RspOutComm_read/1 -> Subsystem/24(MdXX_RspOutComm_Md30_RspOutComm_read)
  MdXX_RspOutComm_Md31_RspOutComm_read/1 -> Subsystem/25(MdXX_RspOutComm_Md31_RspOutComm_read)
  MdXX_RspOutComm_Md32_RspOutComm_read/1 -> Subsystem/26(MdXX_RspOutComm_Md32_RspOutComm_read)
  MdXX_RspOutComm_Md4_RspOutComm_read/1 -> Subsystem/27(MdXX_RspOutComm_Md4_RspOutComm_read)
  MdXX_RspOutComm_Md5_RspOutComm_read/1 -> Subsystem/28(MdXX_RspOutComm_Md5_RspOutComm_read)
  MdXX_RspOutComm_Md6_RspOutComm_read/1 -> Subsystem/29(MdXX_RspOutComm_Md6_RspOutComm_read)
  MdXX_RspOutComm_Md7_RspOutComm_read/1 -> Subsystem/30(MdXX_RspOutComm_Md7_RspOutComm_read)
  MdXX_RspOutComm_Md8_RspOutComm_read/1 -> Subsystem/31(MdXX_RspOutComm_Md8_RspOutComm_read)
  MdXX_RspOutComm_Md9_RspOutComm_read/1 -> Subsystem/32(MdXX_RspOutComm_Md9_RspOutComm_read)
  MdXX_SrcReqTp_Md1_SrcTp_read/1 -> Subsystem/33(MdXX_SrcReqTp_Md1_SrcTp_read)
  MdXX_SrcReqTp_Md10_SrcTp_read/1 -> Subsystem/34(MdXX_SrcReqTp_Md10_SrcTp_read)
  MdXX_SrcReqTp_Md11_SrcTp_read/1 -> Subsystem/35(MdXX_SrcReqTp_Md11_SrcTp_read)
  MdXX_SrcReqTp_Md12_SrcTp_read/1 -> Subsystem/36(MdXX_SrcReqTp_Md12_SrcTp_read)
  MdXX_SrcReqTp_Md13_SrcTp_read/1 -> Subsystem/37(MdXX_SrcReqTp_Md13_SrcTp_read)
  MdXX_SrcReqTp_Md14_SrcTp_read/1 -> Subsystem/38(MdXX_SrcReqTp_Md14_SrcTp_read)
  MdXX_SrcReqTp_Md15_SrcTp_read/1 -> Subsystem/39(MdXX_SrcReqTp_Md15_SrcTp_read)
  MdXX_SrcReqTp_Md16_SrcTp_read/1 -> Subsystem/40(MdXX_SrcReqTp_Md16_SrcTp_read)
  MdXX_SrcReqTp_Md17_SrcTp_read/1 -> Subsystem/41(MdXX_SrcReqTp_Md17_SrcTp_read)
  MdXX_SrcReqTp_Md18_SrcTp_read/1 -> Subsystem/42(MdXX_SrcReqTp_Md18_SrcTp_read)
  MdXX_SrcReqTp_Md19_SrcTp_read/1 -> Subsystem/43(MdXX_SrcReqTp_Md19_SrcTp_read)
  MdXX_SrcReqTp_Md2_SrcTp_read/1 -> Subsystem/44(MdXX_SrcReqTp_Md2_SrcTp_read)
  MdXX_SrcReqTp_Md20_SrcTp_read/1 -> Subsystem/45(MdXX_SrcReqTp_Md20_SrcTp_read)
  MdXX_SrcReqTp_Md21_SrcTp_read/1 -> Subsystem/46(MdXX_SrcReqTp_Md21_SrcTp_read)
  MdXX_SrcReqTp_Md22_SrcTp_read/1 -> Subsystem/47(MdXX_SrcReqTp_Md22_SrcTp_read)
  MdXX_SrcReqTp_Md23_SrcTp_read/1 -> Subsystem/48(MdXX_SrcReqTp_Md23_SrcTp_read)
  MdXX_SrcReqTp_Md24_SrcTp_read/1 -> Subsystem/49(MdXX_SrcReqTp_Md24_SrcTp_read)
  MdXX_SrcReqTp_Md25_SrcTp_read/1 -> Subsystem/50(MdXX_SrcReqTp_Md25_SrcTp_read)
  MdXX_SrcReqTp_Md26_SrcTp_read/1 -> Subsystem/51(MdXX_SrcReqTp_Md26_SrcTp_read)
  MdXX_SrcReqTp_Md27_SrcTp_read/1 -> Subsystem/52(MdXX_SrcReqTp_Md27_SrcTp_read)
  MdXX_SrcReqTp_Md28_SrcTp_read/1 -> Subsystem/53(MdXX_SrcReqTp_Md28_SrcTp_read)
  MdXX_SrcReqTp_Md29_SrcTp_read/1 -> Subsystem/54(MdXX_SrcReqTp_Md29_SrcTp_read)
  MdXX_SrcReqTp_Md3_SrcTp_read/1 -> Subsystem/55(MdXX_SrcReqTp_Md3_SrcTp_read)
  MdXX_SrcReqTp_Md30_SrcTp_read/1 -> Subsystem/56(MdXX_SrcReqTp_Md30_SrcTp_read)
  MdXX_SrcReqTp_Md31_SrcTp_read/1 -> Subsystem/57(MdXX_SrcReqTp_Md31_SrcTp_read)
  MdXX_SrcReqTp_Md32_SrcTp_read/1 -> Subsystem/58(MdXX_SrcReqTp_Md32_SrcTp_read)
  MdXX_SrcReqTp_Md4_SrcTp_read/1 -> Subsystem/59(MdXX_SrcReqTp_Md4_SrcTp_read)
  MdXX_SrcReqTp_Md5_SrcTp_read/1 -> Subsystem/60(MdXX_SrcReqTp_Md5_SrcTp_read)
  MdXX_SrcReqTp_Md6_SrcTp_read/1 -> Subsystem/61(MdXX_SrcReqTp_Md6_SrcTp_read)
  MdXX_SrcReqTp_Md7_SrcTp_read/1 -> Subsystem/62(MdXX_SrcReqTp_Md7_SrcTp_read)
  MdXX_SrcReqTp_Md8_SrcTp_read/1 -> Subsystem/63(MdXX_SrcReqTp_Md8_SrcTp_read)
  MdXX_SrcReqTp_Md9_SrcTp_read/1 -> Subsystem/64(MdXX_SrcReqTp_Md9_SrcTp_read)
  Subsystem/1(IfVeSMSuHMI2L_StMd1_Rsp_Val_write) -> IfVeSMSuHMI2L_StMd1_Rsp_Val_write/1
  Subsystem/2(IfVeSMSuHMI2L_StMd10_Rsp_Val_write) -> IfVeSMSuHMI2L_StMd10_Rsp_Val_write/1
  Subsystem/3(IfVeSMSuHMI2L_StMd11_Rsp_Val_write) -> IfVeSMSuHMI2L_StMd11_Rsp_Val_write/1
  Subsystem/4(IfVeSMSuHMI2L_StMd12_Rsp_Val_write) -> IfVeSMSuHMI2L_StMd12_Rsp_Val_write/1
  Subsystem/5(IfVeSMSuHMI2L_StMd13_Rsp_Val_write) -> IfVeSMSuHMI2L_StMd13_Rsp_Val_write/1
  Subsystem/6(IfVeSMSuHMI2L_StMd14_Rsp_Val_write) -> IfVeSMSuHMI2L_StMd14_Rsp_Val_write/1
  Subsystem/7(IfVeSMSuHMI2L_StMd15_Rsp_Val_write) -> IfVeSMSuHMI2L_StMd15_Rsp_Val_write/1
  Subsystem/8(IfVeSMSuHMI2L_StMd16_Rsp_Val_write) -> IfVeSMSuHMI2L_StMd16_Rsp_Val_write/1
  Subsystem/9(IfVeSMSuHMI2L_StMd17_Rsp_Val_write) -> IfVeSMSuHMI2L_StMd17_Rsp_Val_write/1
  Subsystem/10(IfVeSMSuHMI2L_StMd18_Rsp_Val_write) -> IfVeSMSuHMI2L_StMd18_Rsp_Val_write/1
  Subsystem/11(IfVeSMSuHMI2L_StMd19_Rsp_Val_write) -> IfVeSMSuHMI2L_StMd19_Rsp_Val_write/1
  Subsystem/12(IfVeSMSuHMI2L_StMd2_Rsp_Val_write) -> IfVeSMSuHMI2L_StMd2_Rsp_Val_write/1
  Subsystem/13(IfVeSMSuHMI2L_StMd20_Rsp_Val_write) -> IfVeSMSuHMI2L_StMd20_Rsp_Val_write/1
  Subsystem/14(IfVeSMSuHMI2L_StMd21_Rsp_Val_write) -> IfVeSMSuHMI2L_StMd21_Rsp_Val_write/1
  Subsystem/15(IfVeSMSuHMI2L_StMd22_Rsp_Val_write) -> IfVeSMSuHMI2L_StMd22_Rsp_Val_write/1
  Subsystem/16(IfVeSMSuHMI2L_StMd23_Rsp_Val_write) -> IfVeSMSuHMI2L_StMd23_Rsp_Val_write/1
  Subsystem/17(IfVeSMSuHMI2L_StMd24_Rsp_Val_write) -> IfVeSMSuHMI2L_StMd24_Rsp_Val_write/1
  Subsystem/18(IfVeSMSuHMI2L_StMd25_Rsp_Val_write) -> IfVeSMSuHMI2L_StMd25_Rsp_Val_write/1
  Subsystem/19(IfVeSMSuHMI2L_StMd26_Rsp_Val_write) -> IfVeSMSuHMI2L_StMd26_Rsp_Val_write/1
  Subsystem/20(IfVeSMSuHMI2L_StMd27_Rsp_Val_write) -> IfVeSMSuHMI2L_StMd27_Rsp_Val_write/1
  Subsystem/21(IfVeSMSuHMI2L_StMd28_Rsp_Val_write) -> IfVeSMSuHMI2L_StMd28_Rsp_Val_write/1
  Subsystem/22(IfVeSMSuHMI2L_StMd29_Rsp_Val_write) -> IfVeSMSuHMI2L_StMd29_Rsp_Val_write/1
  Subsystem/23(IfVeSMSuHMI2L_StMd3_Rsp_Val_write) -> IfVeSMSuHMI2L_StMd3_Rsp_Val_write/1
  Subsystem/24(IfVeSMSuHMI2L_StMd30_Rsp_Val_write) -> IfVeSMSuHMI2L_StMd30_Rsp_Val_write/1
  Subsystem/25(IfVeSMSuHMI2L_StMd31_Rsp_Val_write) -> IfVeSMSuHMI2L_StMd31_Rsp_Val_write/1
  Subsystem/26(IfVeSMSuHMI2L_StMd32_Rsp_Val_write) -> IfVeSMSuHMI2L_StMd32_Rsp_Val_write/1
  Subsystem/27(IfVeSMSuHMI2L_StMd4_Rsp_Val_write) -> IfVeSMSuHMI2L_StMd4_Rsp_Val_write/1
  Subsystem/28(IfVeSMSuHMI2L_StMd5_Rsp_Val_write) -> IfVeSMSuHMI2L_StMd5_Rsp_Val_write/1
  Subsystem/29(IfVeSMSuHMI2L_StMd6_Rsp_Val_write) -> IfVeSMSuHMI2L_StMd6_Rsp_Val_write/1
  Subsystem/30(IfVeSMSuHMI2L_StMd7_Rsp_Val_write) -> IfVeSMSuHMI2L_StMd7_Rsp_Val_write/1
  Subsystem/31(IfVeSMSuHMI2L_StMd8_Rsp_Val_write) -> IfVeSMSuHMI2L_StMd8_Rsp_Val_write/1
  Subsystem/32(IfVeSMSuHMI2L_StMd9_Rsp_Val_write) -> IfVeSMSuHMI2L_StMd9_Rsp_Val_write/1

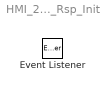
== system HMI_2L_StMdXX_Rsp/HMI_2L_StMdXX_Rsp_Init ==
  Event Listener : EventListener  EventName=reset
